simulink library "TuningHandler"  (R2016b)
settings: Solver=VariableStepAuto  StartTime=0.0  StopTime=10.0  RelTol=1e-3
undefined symbols (not defined in the file or in its folder): sampleTimeSimulink, somanetSyncMode
libraries: ConversionsLibrary x4
settings Model: Creator=Nathan  LastModifiedBy=march

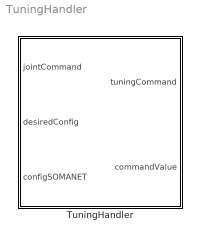
== system TuningHandler ==
  TuningHandler : Subsystem

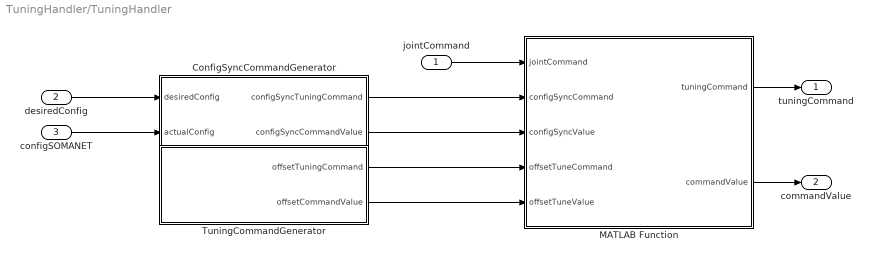
== system TuningHandler/TuningHandler ==
  jointCommand : Inport  OutDataTypeStr=Enum: JointCommand  PortDimensions=1  SampleTime=0.002
  desiredConfig : Inport  Port=2  OutDataTypeStr=Bus: JointControlConfig  PortDimensions=15  SampleTime=0.002
  configSOMANET : Inport  Port=3  OutDataTypeStr=Bus: JointControlConfig  PortDimensions=15  SampleTime=[0.002,0]
  ConfigSyncCommandGenerator : Subsystem
  MATLAB Function : MATLAB Function  TreatAsAtomicUnit=on
  TuningCommandGenerator : Subsystem
  tuningCommand : Outport  PortDimensions=1  SampleTime=[0.002,0]
  commandValue : Outport  Port=2  PortDimensions=1  SampleTime=[0.002,0]
  wires:
  MATLAB Function/1(tuningCommand) -> tuningCommand/1
  desiredConfig/1 -> ConfigSyncCommandGenerator/1(desiredConfig)
  configSOMANET/1 -> ConfigSyncCommandGenerator/2(actualConfig)
  jointCommand/1 -> MATLAB Function/1(jointCommand)
  ConfigSyncCommandGenerator/1(configSyncTuningCommand) -> MATLAB Function/2(configSyncCommand)
  TuningCommandGenerator/1(offsetTuningCommand) -> MATLAB Function/4(offsetTuneCommand)
  TuningCommandGenerator/2(offsetCommandValue) -> MATLAB Function/5(offsetTuneValue)
  ConfigSyncCommandGenerator/2(configSyncCommandValue) -> MATLAB Function/3(configSyncValue)
  MATLAB Function/2(commandValue) -> commandValue/1

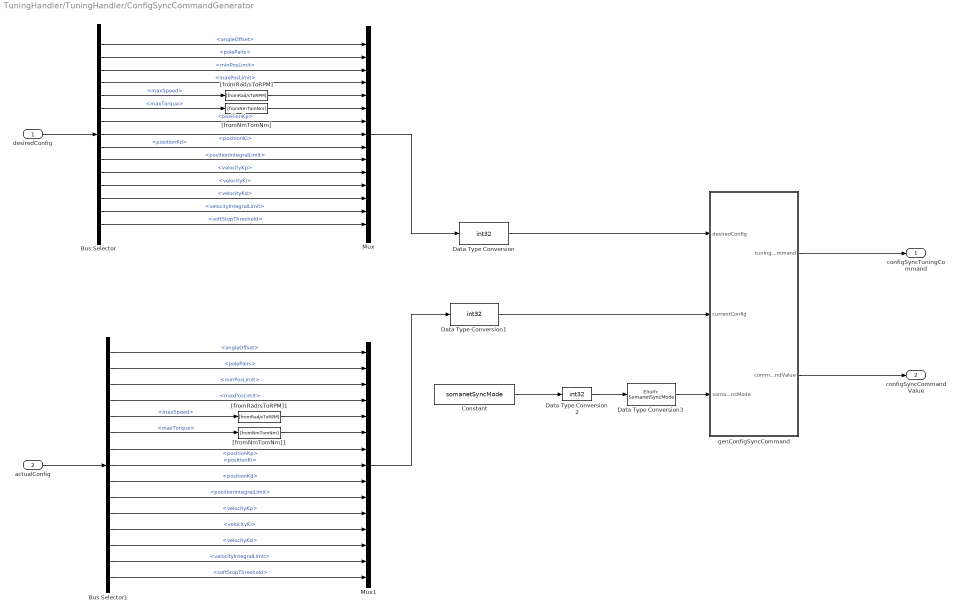
== system TuningHandler/TuningHandler/ConfigSyncCommandGenerator ==
  desiredConfig : Inport
  actualConfig : Inport  Port=2
  Bus Selector : BusSelector  OutputSignals=angleOffset,polePairs,minPosLimit,maxPosLimit,maxSpeed,maxTorque,positionKp,positionKi,positionKd,positionIntegralLimit,velocityKp,velocityKi,velocityKd,velocityIntegralLimit,softStopThreshold
  Bus Selector1 : BusSelector  OutputSignals=angleOffset,polePairs,minPosLimit,maxPosLimit,maxSpeed,maxTorque,positionKp,positionKi,positionKd,positionIntegralLimit,velocityKp,velocityKi,velocityKd,velocityIntegralLimit,softStopThreshold
  Constant : Constant  Value=somanetSyncMode
  Data Type Conversion : DataTypeConversion  OutDataTypeStr=int32  RndMeth=Nearest
  Data Type Conversion1 : DataTypeConversion  OutDataTypeStr=int32  RndMeth=Nearest
  Data Type Conversion2 : DataTypeConversion  OutDataTypeStr=int32
  Data Type Conversion3 : DataTypeConversion  OutDataTypeStr=Enum: SomanetSyncMode
  Mux : Mux  Inputs=15
  Mux1 : Mux  Inputs=15
  "[fromNmTomNm]" : ConversionsLibrary/[fromNmTomNm]
  "[fromNmTomNm]1" : ConversionsLibrary/[fromNmTomNm]
  "[fromRad/sToRPM]" : ConversionsLibrary/[fromRad//sToRPM]
  "[fromRad/sToRPM]1" : ConversionsLibrary/[fromRad//sToRPM]
  genConfigSyncCommand : MATLAB Function  TreatAsAtomicUnit=on  SystemSampleTime=sampleTimeSimulink
  configSyncTuningCommand : Outport
  configSyncCommandValue : Outport  Port=2
  wires:
  Constant/1 -> Data Type Conversion2/1
  Data Type Conversion/1 -> genConfigSyncCommand/1(desiredConfig)
  Bus Selector/3 -> Mux/3  "<minPosLimit>"
  Data Type Conversion1/1 -> genConfigSyncCommand/2(currentConfig)
  genConfigSyncCommand/1(tuningCommand) -> configSyncTuningCommand/1
  Bus Selector1/8 -> Mux1/8  "<positionKi>"
  Bus Selector1/7 -> Mux1/7  "<positionKp>"
  Bus Selector1/5 -> "[fromRad/sToRPM]1"/1  "<maxSpeed>"
  Bus Selector1/4 -> Mux1/4  "<maxPosLimit>"
  Bus Selector1/6 -> "[fromNmTomNm]1"/1  "<maxTorque>"
  Bus Selector1/2 -> Mux1/2  "<polePairs>"
  Bus Selector1/1 -> Mux1/1  "<angleOffset>"
  actualConfig/1 -> Bus Selector1/1
  "[fromRad/sToRPM]"/1 -> Mux/5
  genConfigSyncCommand/2(commandValue) -> configSyncCommandValue/1
  "[fromNmTomNm]1"/1 -> Mux1/6
  Mux1/1 -> Data Type Conversion1/1
  Bus Selector1/14 -> Mux1/14  "<velocityIntegralLimit>"
  Bus Selector1/13 -> Mux1/13  "<velocityKd>"
  desiredConfig/1 -> Bus Selector/1
  Bus Selector1/15 -> Mux1/15  "<softStopThreshold>"
  "[fromNmTomNm]"/1 -> Mux/6
  Mux/1 -> Data Type Conversion/1
  "[fromRad/sToRPM]1"/1 -> Mux1/5
  Bus Selector1/12 -> Mux1/12  "<velocityKi>"
  Bus Selector1/11 -> Mux1/11  "<velocityKp>"
  Bus Selector1/10 -> Mux1/10  "<positionIntegralLimit>"
  Bus Selector1/9 -> Mux1/9  "<positionKd>"
  Bus Selector1/3 -> Mux1/3  "<minPosLimit>"
  Bus Selector/11 -> Mux/11  "<velocityKp>"
  Bus Selector/10 -> Mux/10  "<positionIntegralLimit>"
  Bus Selector/8 -> Mux/8  "<positionKi>"
  Bus Selector/15 -> Mux/15  "<softStopThreshold>"
  Bus Selector/14 -> Mux/14  "<velocityIntegralLimit>"
  Bus Selector/1 -> Mux/1  "<angleOffset>"
  Bus Selector/5 -> "[fromRad/sToRPM]"/1  "<maxSpeed>"
  Bus Selector/6 -> "[fromNmTomNm]"/1  "<maxTorque>"
  Bus Selector/12 -> Mux/12  "<velocityKi>"
  Bus Selector/2 -> Mux/2  "<polePairs>"
  Bus Selector/9 -> Mux/9  "<positionKd>"
  Bus Selector/13 -> Mux/13  "<velocityKd>"
  Bus Selector/7 -> Mux/7  "<positionKp>"
  Bus Selector/4 -> Mux/4  "<maxPosLimit>"
  Data Type Conversion2/1 -> Data Type Conversion3/1
  Data Type Conversion3/1 -> genConfigSyncCommand/3(somanetSyncMode)

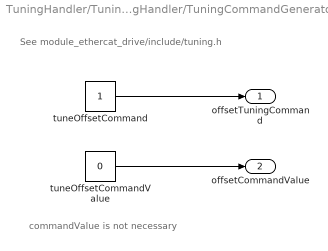
== system TuningHandler/TuningHandler/TuningCommandGenerator ==
  note: commandValue is not necessary
  note: See module_ethercat_drive/include/tuning.h
  tuneOffsetCommand : Constant  OutDataTypeStr=double
  tuneOffsetCommandValue : Constant  Value=0
  offsetTuningCommand : Outport
  offsetCommandValue : Outport  Port=2
  wires:
  tuneOffsetCommand/1 -> offsetTuningCommand/1
  tuneOffsetCommandValue/1 -> offsetCommandValue/1

== matlab function TuningHandler/MATLAB Function ==
  data: jointCommand input; tuningCommand output; configSyncCommand input; configSyncValue input; offsetTuneCommand input; offsetTuneValue input; commandValue output
function [ tuningCommand, commandValue ] = selectTuningCommand( jointCommand, configSyncCommand, configSyncValue, offsetTuneCommand, offsetTuneValue )
% wrapper for selectTuningCommand
[ tuningCommand, commandValue ] = selectTuningCommand( jointCommand, configSyncCommand, configSyncValue, offsetTuneCommand, offsetTuneValue );
end

== matlab function TuningHandler/ConfigSyncCommandGenerator/genConfigSyncCommand ==
  data: desiredConfig input; currentConfig input; tuningCommand output; commandValue output; somanetSyncMode input
function [tuningCommand,commandValue] = genConfigSyncCommand( desiredConfig, currentConfig, somanetSyncMode )
% wrapper for genConfigSyncCommand
[tuningCommand,commandValue] = genConfigSyncCommand( desiredConfig, currentConfig, somanetSyncMode );
end
